simulink model "Current_torque_111"  (R2017b)
settings: Solver=ode45  StartTime=0.0  StopTime=3  MaxStep=1e-4  RelTol=1e-3  EnableMultiTasking=on
libraries: neural x38, fuzblock x6, simulink x1
(part 3 of 3)

== matlab function Current_torque_111/nonliner motor /Permanent Magnet Motor d-q2/Iron loss model/IronLoss ==
  data: omega input; ida output; psi_d input; psi_q input; psi_m input; iqa output; pFe_hy output; pFe_ed output; pFe_ex output; pFe output; Vd input; Vq input; id input; iq input; Rs input
function [ida,iqa,pFe_hy,pFe_ed,pFe_ex,pFe] = IronLoss(omega,psi_d,psi_q,psi_m,Vd,Vq,id,iq,Rs)
%#eml


% Original
% ah=0.306835612;
% ae=0.001287906;
% ax=0.006861992;
% bh=0.209903105;
% be=0.003009911;
% bx=0.013903256;

% Considering build factor 1.5
ah=0.460253418;
ae=0.001931859;
ax=0.010292989;
bh=0.314854657;
be=0.004514867;
bx=0.020854884;

m=3; %number of phases

Vm=omega*sqrt(psi_d^2+psi_q^2);
Vda=-omega*(psi_d-psi_m);

if psi_m~=0
    pFe_hy_oc=ah*(abs(Vm/(2*pi*psi_m)));
    pFe_ed_oc=ae*(abs(Vm/(2*pi*psi_m)))^2;
    pFe_ex_oc=ax*(abs(Vm/(2*pi*psi_m)))^1.5;

    pFe_hy_sc=bh*(abs(Vda/(2*pi*psi_m)));
    pFe_ed_sc=be*(abs(Vda/(2*pi*psi_m)))^2;
    pFe_ex_sc=bx*(abs(Vda/(2*pi*psi_m)))^1.5;
    
    pFe_hy=pFe_hy_oc+pFe_hy_sc;
    pFe_ed=pFe_ed_oc+pFe_ed_sc;
    pFe_ex=pFe_ex_oc+pFe_ex_sc;
    
    pFe_oc=pFe_hy_oc+pFe_ed_oc+pFe_ex_oc;
    pFe_sc=pFe_hy_sc+pFe_ed_sc+pFe_ex_sc;
    pFe=pFe_hy+pFe_ed+pFe_ex;

    if sqrt(psi_d^2+psi_q^2)~=0
        pFe_md=abs(psi_q/sqrt(psi_d^2+psi_q^2))*pFe_oc+pFe_sc;
        pFe_mq=abs(psi_d/sqrt(psi_d^2+psi_q^2))*pFe_oc;
    else
        pFe_md=0.5*pFe_oc+pFe_sc;
        pFe_mq=0.5*pFe_oc;
    end
    
    Vd1=Vd-id*Rs;
    if abs(Vd1)>=0.1
        if (psi_d*iq-psi_q*id)*omega>=0                 %motor
            if id<=0
                ida=id+2/m*abs(pFe_md/Vd1);
            else
                ida=id-2/m*abs(pFe_md/Vd1);
            end
        else                                            %generator
            if id<=0
                ida=id-2/m*abs(pFe_md/Vd1);
            else
                ida=id+2/m*abs(pFe_md/Vd1);
            end          
        end
    else
        ida=id;
    end
    
    Vq1=Vq-iq*Rs;
    if abs(Vq1)>=0.1
        if (psi_d*iq-psi_q*id)*omega>=0                 %motor        
            if iq>=0
                iqa=iq-2/m*abs(pFe_mq/Vq1);
            else
                iqa=iq+2/m*abs(pFe_mq/Vq1);
            end
        else                                            %generator
            if iq>=0
                iqa=iq+2/m*abs(pFe_mq/Vq1);
            else
                iqa=iq-2/m*abs(pFe_mq/Vq1);
            end          
        end
    else
        iqa=iq;
    end


else
    ida=id;
    iqa=iq;
    pFe_hy=0;
    pFe_ed=0;
    pFe_ex=0;
    pFe=0;
end

== matlab function Current_torque_111/voltage limitation/US ==
  data: ud input; us output; uq input
function us = US(ud,uq)
%#codegen
us= (ud^2+uq^2)^0.5+0.01;
